simulink library "halout"  (R2021b)
settings: Solver=VariableStepAuto  StartTime=0.0  StopTime=10.0  RelTol=1e-3
undefined symbols (not defined in the file): C_TASK_5MS_S, FALSE, KHAL_CAN1FD1APS3E2E_flg, KHAL_CAN1FD1APS3TxReq_flg, KHAL_CAN1FD1VCU2E2E_flg, KHAL_CAN1FD1VCU2TxReq_flg, KHAL_CAN1FD1VCU3E2E_flg, KHAL_CAN1FD1VCU3TxReq_flg, KHAL_CAN1TxReq_flg, KHAL_CAN1VMCFCM1E2E_flg, KHAL_CAN1VMCFCM1TxReq_flg, KHAL_CAN2TxReq_flg, KHAL_CAN3FD3VCU1toNIDECTxReq_flg, KHAL_CAN3FD3VCU1TxReq_flg, KHAL_CAN3FD3VCU2E2E_flg, KHAL_CAN3FD3VCU2toNIDECE2E_flg, KHAL_CAN3FD3VCU2toNIDECTxReq_flg, KHAL_CAN3FD3VCU2TxReq_flg, KHAL_CAN3TxReq_flg, KHAL_CAN4FD4CE1000E2E_flg, KHAL_CAN4FD4CE1000TxReq_flg, KHAL_CAN4TxReq_flg, KHAL_CAN5TxReq_flg, KHAL_CAN6FD6APS3E2E_flg, KHAL_CAN6FD6APS3TxReq_flg, KHAL_CAN6FD6VCU2E2E_flg, KHAL_CAN6FD6VCU2TxReq_flg, KHAL_CAN6TxReq_flg, ONE_INT, TRUE, ZERO_INT
libraries: FVT_lib x551, simulink x244
(part 1 of 26)
settings Model: Creator=13168  LastModifiedBy=FVT23136
settings SolverCC: AlgebraicLoopSolver=TrustRegion
settings DataIOCC: SaveFormat=Array  SignalLoggingSaveFormat=ModelDataLogs  ReturnWorkspaceOutputs=off
settings OptimizationCC: BlockReduction=off  BooleanDataType=off
settings DebuggingCC: SaveWithParameterizedLinksMsg=none  UnderspecifiedInitializationDetection=Classic  MergeDetectMultiDrivingBlocksExec=none  SignalResolutionControl=TryResolveAllWithWarning  SFMachineParentedDataDiag=warning
settings HardwareCC: TargetUnknown=on
settings ModelReferenceCC: PropagateSignalLabelsOutOfModel=off
settings ConfigComp: CovMetricSettings=dw  CovSaveCumulativeToWorkspaceVar=on  CovSaveSingleToWorkspaceVar=on

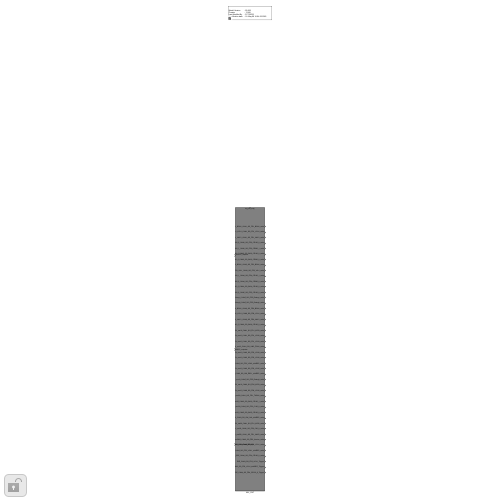
[thumbnail: Simulink's stored preview of the top-level diagram]
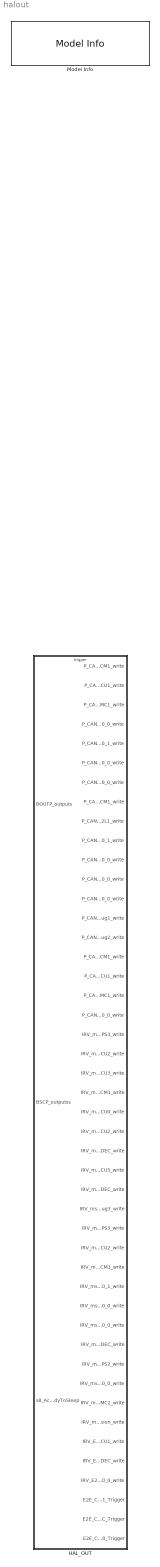
== system halout ==
  HAL_OUT : Subsystem
      settings: RTWSystemCode=Nonreusable function  RTWFcnNameOpts=Use subsystem name  RTWFileNameOpts=Use subsystem name
  Model Info : simulink/Model-Wide Utilities/Model Info  Frame=on  DisplayStringWithTags=|  HorizontalTextAlignment=Left  LeftAlignmentValue=0.02
      | Model Version        : %<ModelVersion>
      | Creator                   : %<Creator>
      | Last Modified By    : %<LastModifiedBy>
      | Modification date    : %<LastModificationDate>

== system halout/HAL_OUT ==
  BOUTP_outputs : Inport  OutDataTypeStr=Bus: BOUTP_outputs
  BSCP_outputss : Inport  Port=2  OutDataTypeStr=Bus: BSCP_outputs
  s8_AcoreReadyToSleep : Inport  Port=3
  trig_hal_out : TriggerPort  TriggerType=function-call  VariantControl=(inherit)
  Bus Selector : BusSelector  OutputSignals=VOUTP_AllCANTxReq_flg
  CAN1 : Subsystem  TreatAsAtomicUnit=on
  CAN2 : Subsystem  TreatAsAtomicUnit=on
  CAN3 : Subsystem  TreatAsAtomicUnit=on
  CAN4 : Subsystem  TreatAsAtomicUnit=on
  CAN5 : Subsystem  TreatAsAtomicUnit=on
  CAN6 : Subsystem  TreatAsAtomicUnit=on
  CAN_Scheduler : Stateflow chart  TreatAsAtomicUnit=on
  Constant : Constant  Value=KHAL_CAN1TxReq_flg
  Constant1 : Constant  Value=KHAL_CAN2TxReq_flg
  Constant2 : Constant  Value=KHAL_CAN3TxReq_flg
  Constant3 : Constant  Value=KHAL_CAN4TxReq_flg
  Constant4 : Constant  Value=KHAL_CAN5TxReq_flg
  Constant5 : Constant  Value=KHAL_CAN6TxReq_flg
  P_CAN1_FD1_BCM1_CAN1_SG_FD1_BCM1_write : Outport  OutDataTypeStr=Bus: DT_CAN1_SG_FD1_BCM1
  P_CAN1_FD1_VCU1_CAN1_SG_FD1_VCU1_write : Outport  Port=2  OutDataTypeStr=Bus: DT_CAN1_SG_FD1_VCU1
  P_CAN1_FD1_VMC1_CAN1_SG_FD1_VMC1_write : Outport  Port=3  OutDataTypeStr=Bus: DT_CAN1_SG_FD1_VMC1
  P_CAN2_FD2_CE100_0_CAN2_SG_FD2_CE100_0_write : Outport  Port=4  OutDataTypeStr=Bus: DT_CAN2_SG_FD2_CE100_0
  P_CAN2_FD2_CE200_1_CAN2_SG_FD2_CE200_1_write : Outport  Port=5  OutDataTypeStr=Bus: DT_CAN2_SG_FD2_CE200_1
  P_CAN2_GW2_CE100_0_CAN2_SG_GW2_CE100_0_write : Outport  Port=6  OutDataTypeStr=Bus: DT_CAN2_SG_GW2_CE100_0
  P_CAN2_GW2_CE200_0_CAN2_SG_GW2_CE200_0_write : Outport  Port=7  OutDataTypeStr=Bus: DT_CAN2_SG_GW2_CE200_0
  P_CAN3_FD3_BCM1_CAN3_SG_FD3_BCM1_write : Outport  Port=8  OutDataTypeStr=Bus: DT_CAN3_SG_FD3_BCM1
  P_CAN3_FD3_V2L1_CAN3_SG_FD3_V2L1_write : Outport  Port=9  OutDataTypeStr=Bus: DT_CAN3_SG_FD3_V2L1
  P_CAN4_FD4_CE100_1_CAN4_SG_FD4_CE100_1_write : Outport  Port=10  OutDataTypeStr=Bus: DT_CAN4_SG_FD4_CE100_1
  P_CAN4_FD4_CE200_0_CAN4_SG_FD4_CE200_0_write : Outport  Port=11  OutDataTypeStr=Bus: DT_CAN4_SG_FD4_CE200_0
  P_CAN4_GW4_CE100_0_CAN4_SG_GW4_CE100_0_write : Outport  Port=12  OutDataTypeStr=Bus: DT_CAN4_SG_GW4_CE100_0
  P_CAN5_FD5_CE100_0_CAN5_SG_FD5_CE100_0_write : Outport  Port=13  OutDataTypeStr=Bus: DT_CAN5_SG_FD5_CE100_0
  P_CAN5_FD5_Debug1_CAN5_SG_FD5_Debug1_write : Outport  Port=14  OutDataTypeStr=Bus: DT_CAN5_SG_FD5_Debug1
  P_CAN5_FD5_Debug2_CAN5_SG_FD5_Debug2_write : Outport  Port=15  OutDataTypeStr=Bus: DT_CAN5_SG_FD5_Debug2
  P_CAN6_FD6_BCM1_CAN6_SG_FD6_BCM1_write : Outport  Port=16  OutDataTypeStr=Bus: DT_CAN6_SG_FD6_BCM1
  P_CAN6_FD6_VCU1_CAN6_SG_FD6_VCU1_write : Outport  Port=17  OutDataTypeStr=Bus: DT_CAN6_SG_FD6_VCU1
  P_CAN6_FD6_VMC1_CAN6_SG_FD6_VMC1_write : Outport  Port=18  OutDataTypeStr=Bus: DT_CAN6_SG_FD6_VMC1
  P_CAN6_GW6_CE100_0_CAN6_SG_GW6_CE100_0_write : Outport  Port=19  OutDataTypeStr=Bus: DT_CAN6_SG_GW6_CE100_0
  IRV_ms10_CAN1_SG_FD1_APS3_write : Outport  Port=20  OutDataTypeStr=Bus: DT_CAN1_SG_FD1_APS3
  IRV_ms10_CAN1_SG_FD1_VCU2_write : Outport  Port=21  OutDataTypeStr=Bus: DT_CAN1_SG_FD1_VCU2
  IRV_ms10_CAN1_SG_FD1_VCU3_write : Outport  Port=22  OutDataTypeStr=Bus: DT_CAN1_SG_FD1_VCU3
  IRV_ms10_CAN1_SG_VMC_FCM1_write : Outport  Port=23  OutDataTypeStr=Bus: DT_CAN1_SG_VMC_FCM1
  IRV_ms10_CAN3_SG_FD3_VCU0_write : Outport  Port=24  OutDataTypeStr=Bus: DT_CAN3_SG_FD3_VCU0
  IRV_ms10_CAN3_SG_FD3_VCU2_write : Outport  Port=25  OutDataTypeStr=Bus: DT_CAN3_SG_FD3_VCU2
  IRV_ms10_CAN3_SG_FD3_VCU2_toNIDEC_write : Outport  Port=26  OutDataTypeStr=Bus: DT_CAN3_SG_FD3_VCU2_toNIDEC
  IRV_ms10_CAN3_SG_FD3_VCU5_write : Outport  Port=27  OutDataTypeStr=Bus: DT_CAN3_SG_FD3_VCU5
  IRV_ms10_CAN3_SG_GW_ESC1_toNIDEC_write : Outport  Port=28  OutDataTypeStr=Bus: DT_CAN3_SG_GW_ESC1_toNIDEC
  IRV_ms10_CAN5_SG_FD5_Debug3_write : Outport  Port=29  OutDataTypeStr=Bus: DT_CAN5_SG_FD5_Debug3
  IRV_ms10_CAN6_SG_FD6_APS3_write : Outport  Port=30  OutDataTypeStr=Bus: DT_CAN6_SG_FD6_APS3
  IRV_ms10_CAN6_SG_FD6_VCU2_write : Outport  Port=31  OutDataTypeStr=Bus: DT_CAN6_SG_FD6_VCU2
  IRV_ms100_CAN1_SG_FD1_THCM1_write : Outport  Port=32  OutDataTypeStr=Bus: DT_CAN1_SG_FD1_THCM1
  IRV_ms100_CAN2_SG_GW2_CE100_1_write : Outport  Port=33  OutDataTypeStr=Bus: DT_CAN2_SG_GW2_CE100_1
  IRV_ms100_CAN3_SG_FD3_C100_0_write : Outport  Port=34  OutDataTypeStr=Bus: DT_CAN3_SG_FD3_C100_0
  IRV_ms100_CAN5_SG_GW5_CE100_0_write : Outport  Port=35  OutDataTypeStr=Bus: DT_CAN5_SG_GW5_CE100_0
  IRV_ms1000_CAN3_SG_GW_IVI6_toNIDEC_write : Outport  Port=36  OutDataTypeStr=Bus: DT_CAN3_SG_GW_IVI6_toNIDEC
  IRV_ms20_CAN1_SG_FD1_APS2_write : Outport  Port=37  OutDataTypeStr=Bus: DT_CAN1_SG_FD1_APS2
  IRV_ms20_CAN2_SG_FD2_C20_0_write : Outport  Port=38  OutDataTypeStr=Bus: DT_CAN2_SG_FD2_C20_0
  IRV_ms500_CAN1_SG_FD1_VMC2_write : Outport  Port=39  OutDataTypeStr=Bus: DT_CAN1_SG_FD1_VMC2
  IRV_ms5000_CAN2_SG_FD2_Version_write : Outport  Port=40  OutDataTypeStr=Bus: DT_CAN2_SG_FD2_Version
  IRV_E2E_CAN3_SG_FD3_VCU1_write : Outport  Port=41  OutDataTypeStr=Bus: DT_CAN3_SG_FD3_VCU1
  IRV_E2E_CAN3_SG_FD3_VCU1_toNIDEC_write : Outport  Port=42  OutDataTypeStr=Bus: DT_CAN3_SG_FD3_VCU1_toNIDEC
  IRV_E2E_CAN4_SG_FD4_CE100_0_write : Outport  Port=43  OutDataTypeStr=Bus: DT_CAN4_SG_FD4_CE100_0
  E2E_CAN3_SG_FD3_VCU1_Trigger : Outport  Port=44
  E2E_CAN3_SG_FD3_VCU1_toNIDEC_Trigger : Outport  Port=45
  E2E_CAN4_SG_FD4_CE100_0_Trigger : Outport  Port=46
  wires:
  BSCP_outputss/1 -> [BSCP_outputs]
  BOUTP_outputs/1 -> [BOUTP_outputs]
  Bus Selector/1 -> CAN_Scheduler/7(VOUTP_ALLCANTxReq_flg)  "<VOUTP_AllCANTxReq_flg>"
  [BOUTP_outputs] -> Bus Selector/1
  Constant1/1 -> CAN_Scheduler/2(KHAL_CAN2TxReq_flg)
  Constant3/1 -> CAN_Scheduler/4(KHAL_CAN4TxReq_flg)
  CAN_Scheduler/1(trig_can1()) -> [trig_can1]
  CAN_Scheduler/2(trig_can2()) -> [trig_can2]
  Constant/1 -> CAN_Scheduler/1(KHAL_CAN1TxReq_flg)
  CAN_Scheduler/4(trig_can4()) -> [trig_can4]
  CAN_Scheduler/5(trig_can5()) -> [trig_can5]
  Constant4/1 -> CAN_Scheduler/5(KHAL_CAN5TxReq_flg)
  Constant2/1 -> CAN_Scheduler/3(KHAL_CAN3TxReq_flg)
  CAN_Scheduler/3(trig_can3()) -> [trig_can3]
  [trig_can1] -> CAN1/Trigger
  [trig_can4] -> CAN4/Trigger
  [trig_can5] -> CAN5/Trigger
  [trig_can2] -> CAN2/Trigger
  Constant5/1 -> CAN_Scheduler/6(KHAL_CAN6TxReq_flg)
  CAN_Scheduler/6(trig_can6()) -> [trig_can6]
  [trig_can6] -> CAN6/Trigger
  [trig_can3] -> CAN3/Trigger
  [BSCP_outputs] -> CAN6/2(BSCP_outputs)
  [BSCP_outputs] -> CAN5/2(BSCP_outputs)
  [BOUTP_outputs] -> CAN5/1(BOUTP_outputs)
  [BOUTP_outputs] -> CAN6/1(BOUTP_outputs)
  CAN4/1(E2E_CAN4_SG_FD4_CE100_0_Trigger) -> E2E_CAN4_SG_FD4_CE100_0_Trigger/1
  [BSCP_outputs] -> CAN3/2(BSCP_outputs)
  CAN3/7(E2E_CAN3_SG_FD3_VCU1_toNIDEC_Trigger) -> E2E_CAN3_SG_FD3_VCU1_toNIDEC_Trigger/1
  [BSCP_outputs] -> CAN2/2(BSCP_outputs)
  [BOUTP_outputs] -> CAN1/1(BOUTP_outputs)
  [BOUTP_outputs] -> CAN3/1(BOUTP_outputs)
  CAN4/2(DT_CAN4_SG_FD4_CE100_0) -> IRV_E2E_CAN4_SG_FD4_CE100_0_write/1
  CAN2/4(DT_CAN2_SG_FD2_Version) -> IRV_ms5000_CAN2_SG_FD2_Version_write/1
  CAN3/8(DT_CAN3_SG_FD3_VCU1_toNIDEC) -> IRV_E2E_CAN3_SG_FD3_VCU1_toNIDEC_write/1
  CAN1/9(DT_CAN1_SG_FD1_VMC2) -> IRV_ms500_CAN1_SG_FD1_VMC2_write/1
  CAN2/1(DT_CAN2_SG_FD2_C20_0) -> IRV_ms20_CAN2_SG_FD2_C20_0_write/1
  CAN1/1(DT_CAN1_SG_FD1_APS2) -> IRV_ms20_CAN1_SG_FD1_APS2_write/1
  CAN3/13(DT_CAN3_SG_GW_IVI6_toNIDEC) -> IRV_ms1000_CAN3_SG_GW_IVI6_toNIDEC_write/1
  CAN5/5(DT_CAN5_SG_GW5_CE100_0) -> IRV_ms100_CAN5_SG_GW5_CE100_0_write/1
  CAN6/4(DT_CAN6_SG_FD6_VCU2) -> IRV_ms10_CAN6_SG_FD6_VCU2_write/1
  CAN5/4(DT_CAN5_SG_FD5_Debug3) -> IRV_ms10_CAN5_SG_FD5_Debug3_write/1
  CAN3/11(DT_CAN3_SG_FD3_VCU5) -> IRV_ms10_CAN3_SG_FD3_VCU5_write/1
  CAN3/12(DT_CAN3_SG_GW_ESC1_toNIDEC) -> IRV_ms10_CAN3_SG_GW_ESC1_toNIDEC_write/1
  CAN2/6(DT_CAN2_SG_GW2_CE100_1) -> IRV_ms100_CAN2_SG_GW2_CE100_1_write/1
  CAN3/10(DT_CAN3_SG_FD3_VCU2_toNIDEC) -> IRV_ms10_CAN3_SG_FD3_VCU2_toNIDEC_write/1
  CAN3/9(DT_CAN3_SG_FD3_VCU2) -> IRV_ms10_CAN3_SG_FD3_VCU2_write/1
  CAN3/4(DT_CAN3_SG_FD3_VCU0) -> IRV_ms10_CAN3_SG_FD3_VCU0_write/1
  CAN1/7(DT_CAN1_SG_FD1_VCU3) -> IRV_ms10_CAN1_SG_FD1_VCU3_write/1
  CAN1/10(DT_CAN1_SG_VMC_FCM1) -> IRV_ms10_CAN1_SG_VMC_FCM1_write/1
  CAN6/5(DT_CAN6_SG_FD6_VMC1) -> P_CAN6_FD6_VMC1_CAN6_SG_FD6_VMC1_write/1
  CAN3/2(DT_CAN3_SG_FD3_C100_0) -> IRV_ms100_CAN3_SG_FD3_C100_0_write/1
  CAN3/5(E2E_CAN3_SG_FD3_VCU1_Trigger) -> E2E_CAN3_SG_FD3_VCU1_Trigger/1
  CAN6/6(DT_CAN6_SG_GW6_CE100_0) -> P_CAN6_GW6_CE100_0_CAN6_SG_GW6_CE100_0_write/1
  CAN1/6(DT_CAN1_SG_FD1_VCU2) -> IRV_ms10_CAN1_SG_FD1_VCU2_write/1
  CAN6/3(DT_CAN6_SG_FD6_VCU1) -> P_CAN6_FD6_VCU1_CAN6_SG_FD6_VCU1_write/1
  CAN6/2(DT_CAN6_SG_FD6_BCM1) -> P_CAN6_FD6_BCM1_CAN6_SG_FD6_BCM1_write/1
  CAN5/2(DT_CAN5_SG_FD5_Debug1) -> P_CAN5_FD5_Debug1_CAN5_SG_FD5_Debug1_write/1
  s8_AcoreReadyToSleep/1 -> CAN3/3(s8_AcoreReadyToSleep)
  CAN5/3(DT_CAN5_SG_FD5_Debug2) -> P_CAN5_FD5_Debug2_CAN5_SG_FD5_Debug2_write/1
  CAN5/1(DT_CAN5_SG_FD5_CE100_0) -> P_CAN5_FD5_CE100_0_CAN5_SG_FD5_CE100_0_write/1
  [BOUTP_outputs] -> CAN4/1(BOUTP_outputs)
  CAN4/5(DT_CAN4_SG_GW4_CE100_0) -> P_CAN4_GW4_CE100_0_CAN4_SG_GW4_CE100_0_write/1
  CAN4/3(DT_CAN4_SG_FD4_CE100_1) -> P_CAN4_FD4_CE100_1_CAN4_SG_FD4_CE100_1_write/1
  CAN4/4(DT_CAN4_SG_FD4_CE200_0) -> P_CAN4_FD4_CE200_0_CAN4_SG_FD4_CE200_0_write/1
  CAN3/3(DT_CAN3_SG_FD3_V2L1) -> P_CAN3_FD3_V2L1_CAN3_SG_FD3_V2L1_write/1
  CAN1/4(DT_CAN1_SG_FD1_THCM1) -> IRV_ms100_CAN1_SG_FD1_THCM1_write/1
  CAN3/1(DT_CAN3_SG_FD3_BCM1) -> P_CAN3_FD3_BCM1_CAN3_SG_FD3_BCM1_write/1
  CAN2/7(DT_CAN2_SG_GW2_CE200_0) -> P_CAN2_GW2_CE200_0_CAN2_SG_GW2_CE200_0_write/1
  CAN1/3(DT_CAN1_SG_FD1_BCM1) -> P_CAN1_FD1_BCM1_CAN1_SG_FD1_BCM1_write/1
  CAN2/5(DT_CAN2_SG_GW2_CE100_0) -> P_CAN2_GW2_CE100_0_CAN2_SG_GW2_CE100_0_write/1
  CAN1/8(DT_CAN1_SG_FD1_VMC1) -> P_CAN1_FD1_VMC1_CAN1_SG_FD1_VMC1_write/1
  CAN1/2(DT_CAN1_SG_FD1_APS3) -> IRV_ms10_CAN1_SG_FD1_APS3_write/1
  [BOUTP_outputs] -> CAN2/1(BOUTP_outputs)
  CAN2/2(DT_CAN2_SG_FD2_CE100_0) -> P_CAN2_FD2_CE100_0_CAN2_SG_FD2_CE100_0_write/1
  CAN6/1(DT_CAN6_SG_FD6_APS3) -> IRV_ms10_CAN6_SG_FD6_APS3_write/1
  CAN1/5(DT_CAN1_SG_FD1_VCU1) -> P_CAN1_FD1_VCU1_CAN1_SG_FD1_VCU1_write/1
  [BSCP_outputs] -> CAN4/2(BSCP_outputs)
  CAN3/6(DT_CAN3_SG_FD3_VCU1) -> IRV_E2E_CAN3_SG_FD3_VCU1_write/1
  CAN2/3(DT_CAN2_SG_FD2_CE200_1) -> P_CAN2_FD2_CE200_1_CAN2_SG_FD2_CE200_1_write/1
  [BSCP_outputs] -> CAN1/2(BSCP_outputs)

== system halout/HAL_OUT/CAN1 ==
  BOUTP_outputs : Inport  OutDataTypeStr=Bus: BOUTP_outputs
  BSCP_outputs : Inport  Port=2  OutDataTypeStr=Bus: BSCP_outputs
  Trigger : TriggerPort  TriggerType=function-call  VariantControl=(inherit)
  Constant : Constant  Value=KHAL_CAN1FD1APS3TxReq_flg
  Constant1 : Constant  Value=KHAL_CAN1FD1VCU2TxReq_flg
  Constant2 : Constant  Value=KHAL_CAN1FD1VCU3TxReq_flg
  Constant3 : Constant  Value=KHAL_CAN1VMCFCM1TxReq_flg
  FD1_APS2_0x210 : Subsystem
  FD1_APS3_0x238 : Subsystem  TreatAsAtomicUnit=on
  FD1_APS3_Tx : Subsystem  AncestorBlock=FVT_lib/hal/MsgTxController  mask{CycleTime=10}
      mask prompts: CycleTime "MsgCycleTime_ms"
      mask help: MeasumentTrigerTime
      mask Display: fprintf('Tx Method: Cycle\nMsg Cycletime ms: %3.0f', CycleTime);
  FD1_BCM1_0x216 : Subsystem
  FD1_THCM1_0x182 : Subsystem
  FD1_VCU1_0x116 : Subsystem
  FD1_VCU2_0x154 : Subsystem  TreatAsAtomicUnit=on
  FD1_VCU2_Tx : Subsystem  AncestorBlock=FVT_lib/hal/MsgTxController  mask{CycleTime=10}
      mask prompts: CycleTime "MsgCycleTime_ms"
      mask help: MeasumentTrigerTime
      mask Display: fprintf('Tx Method: Cycle\nMsg Cycletime ms: %3.0f', CycleTime);
  FD1_VCU3_0x159 : Subsystem  TreatAsAtomicUnit=on
  FD1_VCU3_Tx : Subsystem  AncestorBlock=FVT_lib/hal/MsgTxController  mask{CycleTime=10}
      mask prompts: CycleTime "MsgCycleTime_ms"
      mask help: MeasumentTrigerTime
      mask Display: fprintf('Tx Method: Cycle\nMsg Cycletime ms: %3.0f', CycleTime);
  FD1_VMC1_0x17F : Subsystem
  FD1_VMC2_0x77 : Subsystem
  VMC_FCM1_0x172 : Subsystem  TreatAsAtomicUnit=on
  VMC_FCM1_Tx : Subsystem  AncestorBlock=FVT_lib/hal/MsgTxController  mask{CycleTime=10}
      mask prompts: CycleTime "MsgCycleTime_ms"
      mask help: MeasumentTrigerTime
      mask Display: fprintf('Tx Method: Cycle\nMsg Cycletime ms: %3.0f', CycleTime);
  DT_CAN1_SG_FD1_APS2 : Outport  OutDataTypeStr=Bus: DT_CAN1_SG_FD1_APS2
  DT_CAN1_SG_FD1_APS3 : Outport  Port=2  OutDataTypeStr=Bus: DT_CAN1_SG_FD1_APS3
  DT_CAN1_SG_FD1_BCM1 : Outport  Port=3  OutDataTypeStr=Bus: DT_CAN1_SG_FD1_BCM1
  DT_CAN1_SG_FD1_THCM1 : Outport  Port=4  OutDataTypeStr=Bus: DT_CAN1_SG_FD1_THCM1
  DT_CAN1_SG_FD1_VCU1 : Outport  Port=5  OutDataTypeStr=Bus: DT_CAN1_SG_FD1_VCU1
  DT_CAN1_SG_FD1_VCU2 : Outport  Port=6  OutDataTypeStr=Bus: DT_CAN1_SG_FD1_VCU2
  DT_CAN1_SG_FD1_VCU3 : Outport  Port=7  OutDataTypeStr=Bus: DT_CAN1_SG_FD1_VCU3
  DT_CAN1_SG_FD1_VMC1 : Outport  Port=8  OutDataTypeStr=Bus: DT_CAN1_SG_FD1_VMC1
  DT_CAN1_SG_FD1_VMC2 : Outport  Port=9  OutDataTypeStr=Bus: DT_CAN1_SG_FD1_VMC2
  DT_CAN1_SG_VMC_FCM1 : Outport  Port=10  OutDataTypeStr=Bus: DT_CAN1_SG_VMC_FCM1
  wires:
  BOUTP_outputs/1 -> [BOUTP_outputs]
  BSCP_outputs/1 -> [BSCP_outputs]
  [BSCP_outputs] -> FD1_APS2_0x210/1(BSCP_outputs)
  [BOUTP_outputs] -> FD1_APS2_0x210/2(BOUTP_outputs)
  FD1_APS2_0x210/1(FD1_APS2) -> DT_CAN1_SG_FD1_APS2/1
  [BSCP_outputs] -> FD1_APS3_0x238/1(BSCP_outputs)
  [BOUTP_outputs] -> FD1_APS3_0x238/2(BOUTP_outputs)
  FD1_APS3_Tx/1(TxTrigger) -> FD1_APS3_0x238/Trigger
  Constant/1 -> FD1_APS3_Tx/1(TxReq)
  FD1_APS3_0x238/1(FD1_APS3) -> DT_CAN1_SG_FD1_APS3/1
  [BSCP_outputs] -> FD1_BCM1_0x216/1(BSCP_outputs)
  [BOUTP_outputs] -> FD1_BCM1_0x216/2(BOUTP_outputs)
  FD1_BCM1_0x216/1(FD1_BCM1) -> DT_CAN1_SG_FD1_BCM1/1
  [BSCP_outputs] -> FD1_THCM1_0x182/1(BSCP_outputs)
  [BOUTP_outputs] -> FD1_THCM1_0x182/2(BOUTP_outputs)
  FD1_THCM1_0x182/1(FD1_THCM1) -> DT_CAN1_SG_FD1_THCM1/1
  [BSCP_outputs] -> FD1_VCU1_0x116/1(BSCP_outputs)
  [BOUTP_outputs] -> FD1_VCU1_0x116/2(BOUTP_outputs)
  FD1_VCU1_0x116/1(FD1_VCU1) -> DT_CAN1_SG_FD1_VCU1/1
  [BSCP_outputs] -> FD1_VCU2_0x154/1(BSCP_outputs)
  [BOUTP_outputs] -> FD1_VCU2_0x154/2(BOUTP_outputs)
  FD1_VCU2_Tx/1(TxTrigger) -> FD1_VCU2_0x154/Trigger
  Constant1/1 -> FD1_VCU2_Tx/1(TxReq)
  FD1_VCU2_0x154/1(FD1_VCU2) -> DT_CAN1_SG_FD1_VCU2/1
  [BSCP_outputs] -> FD1_VCU3_0x159/1(BSCP_outputs)
  [BOUTP_outputs] -> FD1_VCU3_0x159/2(BOUTP_outputs)
  FD1_VCU3_Tx/1(TxTrigger) -> FD1_VCU3_0x159/Trigger
  Constant2/1 -> FD1_VCU3_Tx/1(TxReq)
  FD1_VCU3_0x159/1(FD1_VCU3) -> DT_CAN1_SG_FD1_VCU3/1
  [BSCP_outputs] -> FD1_VMC1_0x17F/1(BSCP_outputs)
  [BOUTP_outputs] -> FD1_VMC1_0x17F/2(BOUTP_outputs)
  FD1_VMC1_0x17F/1(FD1_VMC1) -> DT_CAN1_SG_FD1_VMC1/1
  [BSCP_outputs] -> FD1_VMC2_0x77/1(BSCP_outputs)
  [BOUTP_outputs] -> FD1_VMC2_0x77/2(BOUTP_outputs)
  FD1_VMC2_0x77/1(FD1_VMC2) -> DT_CAN1_SG_FD1_VMC2/1
  [BSCP_outputs] -> VMC_FCM1_0x172/1(BSCP_outputs)
  [BOUTP_outputs] -> VMC_FCM1_0x172/2(BOUTP_outputs)
  VMC_FCM1_Tx/1(TxTrigger) -> VMC_FCM1_0x172/Trigger
  Constant3/1 -> VMC_FCM1_Tx/1(TxReq)
  VMC_FCM1_0x172/1(VMC_FCM1) -> DT_CAN1_SG_VMC_FCM1/1

== system halout/HAL_OUT/CAN2 ==
  BOUTP_outputs : Inport  OutDataTypeStr=Bus: BOUTP_outputs
  BSCP_outputs : Inport  Port=2  OutDataTypeStr=Bus: BSCP_outputs
  Trigger : TriggerPort  TriggerType=function-call  VariantControl=(inherit)
  FD2_C20_0_0x210 : Subsystem
  FD2_CE100_0_0x117 : Subsystem
  FD2_CE200_1_0x435 : Subsystem
  FD2_Version_0x3C3 : Subsystem
  GW2_CE100_0_0x1C2 : Subsystem
  GW2_CE100_1_0x357 : Subsystem
  GW2_CE200_0_0x174 : Subsystem
  DT_CAN2_SG_FD2_C20_0 : Outport  OutDataTypeStr=Bus: DT_CAN2_SG_FD2_C20_0
  DT_CAN2_SG_FD2_CE100_0 : Outport  Port=2  OutDataTypeStr=Bus: DT_CAN2_SG_FD2_CE100_0
  DT_CAN2_SG_FD2_CE200_1 : Outport  Port=3  OutDataTypeStr=Bus: DT_CAN2_SG_FD2_CE200_1
  DT_CAN2_SG_FD2_Version : Outport  Port=4  OutDataTypeStr=Bus: DT_CAN2_SG_FD2_Version
  DT_CAN2_SG_GW2_CE100_0 : Outport  Port=5  OutDataTypeStr=Bus: DT_CAN2_SG_GW2_CE100_0
  DT_CAN2_SG_GW2_CE100_1 : Outport  Port=6  OutDataTypeStr=Bus: DT_CAN2_SG_GW2_CE100_1
  DT_CAN2_SG_GW2_CE200_0 : Outport  Port=7  OutDataTypeStr=Bus: DT_CAN2_SG_GW2_CE200_0
  wires:
  BOUTP_outputs/1 -> [BOUTP_outputs]
  BSCP_outputs/1 -> [BSCP_outputs]
  [BSCP_outputs] -> FD2_C20_0_0x210/1(BSCP_outputs)
  [BOUTP_outputs] -> FD2_C20_0_0x210/2(BOUTP_outputs)
  FD2_C20_0_0x210/1(FD2_C20_0) -> DT_CAN2_SG_FD2_C20_0/1
  [BSCP_outputs] -> FD2_CE100_0_0x117/1(BSCP_outputs)
  [BOUTP_outputs] -> FD2_CE100_0_0x117/2(BOUTP_outputs)
  FD2_CE100_0_0x117/1(FD2_CE100_0) -> DT_CAN2_SG_FD2_CE100_0/1
  [BSCP_outputs] -> FD2_CE200_1_0x435/1(BSCP_outputs)
  [BOUTP_outputs] -> FD2_CE200_1_0x435/2(BOUTP_outputs)
  FD2_CE200_1_0x435/1(FD2_CE200_1) -> DT_CAN2_SG_FD2_CE200_1/1
  [BSCP_outputs] -> FD2_Version_0x3C3/1(BSCP_outputs)
  [BOUTP_outputs] -> FD2_Version_0x3C3/2(BOUTP_outputs)
  FD2_Version_0x3C3/1(FD2_Version) -> DT_CAN2_SG_FD2_Version/1
  [BSCP_outputs] -> GW2_CE100_0_0x1C2/1(BSCP_outputs)
  [BOUTP_outputs] -> GW2_CE100_0_0x1C2/2(BOUTP_outputs)
  GW2_CE100_0_0x1C2/1(GW2_CE100_0) -> DT_CAN2_SG_GW2_CE100_0/1
  [BSCP_outputs] -> GW2_CE100_1_0x357/1(BSCP_outputs)
  [BOUTP_outputs] -> GW2_CE100_1_0x357/2(BOUTP_outputs)
  GW2_CE100_1_0x357/1(GW2_CE100_1) -> DT_CAN2_SG_GW2_CE100_1/1
  [BSCP_outputs] -> GW2_CE200_0_0x174/1(BSCP_outputs)
  [BOUTP_outputs] -> GW2_CE200_0_0x174/2(BOUTP_outputs)
  GW2_CE200_0_0x174/1(GW2_CE200_0) -> DT_CAN2_SG_GW2_CE200_0/1

== system halout/HAL_OUT/CAN3 ==
  BOUTP_outputs : Inport  OutDataTypeStr=Bus: BOUTP_outputs
  BSCP_outputs : Inport  Port=2  OutDataTypeStr=Bus: BSCP_outputs
  s8_AcoreReadyToSleep : Inport  Port=3
  Trigger : TriggerPort  TriggerType=function-call  VariantControl=(inherit)
  Constant : Constant  Value=KHAL_CAN3FD3VCU1TxReq_flg
  Constant1 : Constant  Value=KHAL_CAN3FD3VCU1toNIDECTxReq_flg
  Constant2 : Constant  Value=KHAL_CAN3FD3VCU2TxReq_flg
  Constant3 : Constant  Value=KHAL_CAN3FD3VCU2toNIDECTxReq_flg
  FD3_BCM1_0x216 : Subsystem
  FD3_C100_0_0x182 : Subsystem
  FD3_V2L1_0x374 : Subsystem
  FD3_VCU0_0x1F0 : Subsystem
  FD3_VCU1_0x115 : Subsystem
  FD3_VCU1_Tx : Subsystem  AncestorBlock=FVT_lib/hal/MsgTxController_CE  mask{CycleTime=100}
      mask prompts: CycleTime "MsgCycleTime_ms"
      mask help: MeasumentTrigerTime
      mask Display: fprintf('Tx Method: CE\nMsg Cycletime ms: %3.0f', CycleTime);
  FD3_VCU1_toNIDEC_0x116 : Subsystem
  FD3_VCU1_toNIDEC_Tx : Subsystem  AncestorBlock=FVT_lib/hal/MsgTxController_CE  mask{CycleTime=100}
      mask prompts: CycleTime "MsgCycleTime_ms"
      mask help: MeasumentTrigerTime
      mask Display: fprintf('Tx Method: CE\nMsg Cycletime ms: %3.0f', CycleTime);
  FD3_VCU2_0x153 : Subsystem  TreatAsAtomicUnit=on
  FD3_VCU2_Tx : Subsystem  AncestorBlock=FVT_lib/hal/MsgTxController  mask{CycleTime=10}
      mask prompts: CycleTime "MsgCycleTime_ms"
      mask help: MeasumentTrigerTime
      mask Display: fprintf('Tx Method: Cycle\nMsg Cycletime ms: %3.0f', CycleTime);
  FD3_VCU2_toNIDEC_0x154 : Subsystem  TreatAsAtomicUnit=on
  FD3_VCU2_toNIDEC_Tx : Subsystem  AncestorBlock=FVT_lib/hal/MsgTxController  mask{CycleTime=10}
      mask prompts: CycleTime "MsgCycleTime_ms"
      mask help: MeasumentTrigerTime
      mask Display: fprintf('Tx Method: Cycle\nMsg Cycletime ms: %3.0f', CycleTime);
  FD3_VCU5_0x155 : Subsystem
  GW_ESC1_toNIDEC_0x152 : Subsystem
  GW_IVI6_toNIDEC_0x49F : Subsystem
  DT_CAN3_SG_FD3_BCM1 : Outport  OutDataTypeStr=Bus: DT_CAN3_SG_FD3_BCM1
  DT_CAN3_SG_FD3_C100_0 : Outport  Port=2  OutDataTypeStr=Bus: DT_CAN3_SG_FD3_C100_0
  DT_CAN3_SG_FD3_V2L1 : Outport  Port=3  OutDataTypeStr=Bus: DT_CAN3_SG_FD3_V2L1
  DT_CAN3_SG_FD3_VCU0 : Outport  Port=4  OutDataTypeStr=Bus: DT_CAN3_SG_FD3_VCU0
  E2E_CAN3_SG_FD3_VCU1_Trigger : Outport  Port=5
  DT_CAN3_SG_FD3_VCU1 : Outport  Port=6  OutDataTypeStr=Bus: DT_CAN3_SG_FD3_VCU1
  E2E_CAN3_SG_FD3_VCU1_toNIDEC_Trigger : Outport  Port=7
  DT_CAN3_SG_FD3_VCU1_toNIDEC : Outport  Port=8  OutDataTypeStr=Bus: DT_CAN3_SG_FD3_VCU1_toNIDEC
  DT_CAN3_SG_FD3_VCU2 : Outport  Port=9  OutDataTypeStr=Bus: DT_CAN3_SG_FD3_VCU2
  DT_CAN3_SG_FD3_VCU2_toNIDEC : Outport  Port=10  OutDataTypeStr=Bus: DT_CAN3_SG_FD3_VCU2_toNIDEC
  DT_CAN3_SG_FD3_VCU5 : Outport  Port=11  OutDataTypeStr=Bus: DT_CAN3_SG_FD3_VCU5
  DT_CAN3_SG_GW_ESC1_toNIDEC : Outport  Port=12  OutDataTypeStr=Bus: DT_CAN3_SG_GW_ESC1_toNIDEC
  DT_CAN3_SG_GW_IVI6_toNIDEC : Outport  Port=13  OutDataTypeStr=Bus: DT_CAN3_SG_GW_IVI6_toNIDEC
  wires:
  BOUTP_outputs/1 -> [BOUTP_outputs]
  BSCP_outputs/1 -> [BSCP_outputs]
  [BSCP_outputs] -> FD3_BCM1_0x216/1(BSCP_outputs)
  [BOUTP_outputs] -> FD3_BCM1_0x216/2(BOUTP_outputs)
  FD3_BCM1_0x216/1(FD3_BCM1) -> DT_CAN3_SG_FD3_BCM1/1
  [BSCP_outputs] -> FD3_C100_0_0x182/1(BSCP_outputs)
  [BOUTP_outputs] -> FD3_C100_0_0x182/2(BOUTP_outputs)
  FD3_C100_0_0x182/1(FD3_C100_0) -> DT_CAN3_SG_FD3_C100_0/1
  [BSCP_outputs] -> FD3_V2L1_0x374/1(BSCP_outputs)
  [BOUTP_outputs] -> FD3_V2L1_0x374/2(BOUTP_outputs)
  FD3_V2L1_0x374/1(FD3_V2L1) -> DT_CAN3_SG_FD3_V2L1/1
  [BSCP_outputs] -> FD3_VCU0_0x1F0/1(BSCP_outputs)
  [BOUTP_outputs] -> FD3_VCU0_0x1F0/2(BOUTP_outputs)
  FD3_VCU0_0x1F0/1(FD3_VCU0) -> DT_CAN3_SG_FD3_VCU0/1
  [BSCP_outputs] -> FD3_VCU1_0x115/1(BSCP_outputs)
  [BOUTP_outputs] -> FD3_VCU1_0x115/2(BOUTP_outputs)
  FD3_VCU1_Tx/1(TxTrigger) -> E2E_CAN3_SG_FD3_VCU1_Trigger/1
  Constant/1 -> FD3_VCU1_Tx/1(TxReq)
  [BSCP_outputs] -> FD3_VCU1_Tx/2(BSCP_outputs)
  [BOUTP_outputs] -> FD3_VCU1_Tx/3(BOUTP_outputs)
  FD3_VCU1_0x115/1(FD3_VCU1) -> DT_CAN3_SG_FD3_VCU1/1
  [BSCP_outputs] -> FD3_VCU1_toNIDEC_0x116/1(BSCP_outputs)
  [BOUTP_outputs] -> FD3_VCU1_toNIDEC_0x116/2(BOUTP_outputs)
  FD3_VCU1_toNIDEC_Tx/1(TxTrigger) -> E2E_CAN3_SG_FD3_VCU1_toNIDEC_Trigger/1
  Constant1/1 -> FD3_VCU1_toNIDEC_Tx/1(TxReq)
  [BSCP_outputs] -> FD3_VCU1_toNIDEC_Tx/2(BSCP_outputs)
  [BOUTP_outputs] -> FD3_VCU1_toNIDEC_Tx/3(BOUTP_outputs)
  FD3_VCU1_toNIDEC_0x116/1(FD3_VCU1_toNIDEC) -> DT_CAN3_SG_FD3_VCU1_toNIDEC/1
  [BSCP_outputs] -> FD3_VCU2_0x153/1(BSCP_outputs)
  [BOUTP_outputs] -> FD3_VCU2_0x153/2(BOUTP_outputs)
  FD3_VCU2_Tx/1(TxTrigger) -> FD3_VCU2_0x153/Trigger
  Constant2/1 -> FD3_VCU2_Tx/1(TxReq)
  FD3_VCU2_0x153/1(FD3_VCU2) -> DT_CAN3_SG_FD3_VCU2/1
  [BSCP_outputs] -> FD3_VCU2_toNIDEC_0x154/1(BSCP_outputs)
  [BOUTP_outputs] -> FD3_VCU2_toNIDEC_0x154/2(BOUTP_outputs)
  FD3_VCU2_toNIDEC_Tx/1(TxTrigger) -> FD3_VCU2_toNIDEC_0x154/Trigger
  Constant3/1 -> FD3_VCU2_toNIDEC_Tx/1(TxReq)
  FD3_VCU2_toNIDEC_0x154/1(FD3_VCU2_toNIDEC) -> DT_CAN3_SG_FD3_VCU2_toNIDEC/1
  [BSCP_outputs] -> FD3_VCU5_0x155/1(BSCP_outputs)
  [BOUTP_outputs] -> FD3_VCU5_0x155/2(BOUTP_outputs)
  FD3_VCU5_0x155/1(FD3_VCU5) -> DT_CAN3_SG_FD3_VCU5/1
  [BSCP_outputs] -> GW_ESC1_toNIDEC_0x152/1(BSCP_outputs)
  [BOUTP_outputs] -> GW_ESC1_toNIDEC_0x152/2(BOUTP_outputs)
  GW_ESC1_toNIDEC_0x152/1(GW_ESC1_toNIDEC) -> DT_CAN3_SG_GW_ESC1_toNIDEC/1
  [BSCP_outputs] -> GW_IVI6_toNIDEC_0x49F/1(BSCP_outputs)
  [BOUTP_outputs] -> GW_IVI6_toNIDEC_0x49F/2(BOUTP_outputs)
  GW_IVI6_toNIDEC_0x49F/1(GW_IVI6_toNIDEC) -> DT_CAN3_SG_GW_IVI6_toNIDEC/1
  s8_AcoreReadyToSleep/1 -> FD3_VCU0_0x1F0/3(s8_AcoreReadyToSleep)

== system halout/HAL_OUT/CAN4 ==
  BOUTP_outputs : Inport  OutDataTypeStr=Bus: BOUTP_outputs
  BSCP_outputs : Inport  Port=2  OutDataTypeStr=Bus: BSCP_outputs
  Trigger : TriggerPort  TriggerType=function-call  VariantControl=(inherit)
  Constant : Constant  Value=KHAL_CAN4FD4CE1000TxReq_flg
  Detect Change : simulink/Logic and Bit Operations/Detect Change  vinit=0  OutDataTypeStr=boolean
  FD4_CE100_0_0x116 : Subsystem  TreatAsAtomicUnit=on
  FD4_CE100_0_Tx : Subsystem  AncestorBlock=FVT_lib/hal/MsgTxController_CE  mask{CycleTime=100}
      mask prompts: CycleTime "MsgCycleTime_ms"
      mask help: MeasumentTrigerTime
      mask Display: fprintf('Tx Method: CE\nMsg Cycletime ms: %3.0f', CycleTime);
  FD4_CE100_1_0x182 : Subsystem
  FD4_CE200_0_0x217 : Subsystem
  Function-Call Subsystem : Subsystem  TreatAsAtomicUnit=on
  GW4_CE100_0_0x253 : Subsystem
  Unit Delay : UnitDelay  SampleTime=-1  HasFrameUpgradeWarning=on
  E2E_CAN4_SG_FD4_CE100_0_Trigger : Outport
  DT_CAN4_SG_FD4_CE100_0 : Outport  Port=2  OutDataTypeStr=Bus: DT_CAN4_SG_FD4_CE100_0
  DT_CAN4_SG_FD4_CE100_1 : Outport  Port=3  OutDataTypeStr=Bus: DT_CAN4_SG_FD4_CE100_1
  DT_CAN4_SG_FD4_CE200_0 : Outport  Port=4  OutDataTypeStr=Bus: DT_CAN4_SG_FD4_CE200_0
  DT_CAN4_SG_GW4_CE100_0 : Outport  Port=5  OutDataTypeStr=Bus: DT_CAN4_SG_GW4_CE100_0
  wires:
  BOUTP_outputs/1 -> [BOUTP_outputs]
  BSCP_outputs/1 -> [BSCP_outputs]
  [BSCP_outputs] -> FD4_CE100_0_0x116/1(BSCP_outputs)
  [BOUTP_outputs] -> FD4_CE100_0_0x116/2(BOUTP_outputs)
  Constant/1 -> FD4_CE100_0_Tx/1(TxReq)
  [BSCP_outputs] -> FD4_CE100_0_Tx/2(BSCP_outputs)
  [BOUTP_outputs] -> FD4_CE100_0_Tx/3(BOUTP_outputs)
  FD4_CE100_0_0x116/1(FD4_CE100_0) -> DT_CAN4_SG_FD4_CE100_0/1
  [BSCP_outputs] -> FD4_CE100_1_0x182/1(BSCP_outputs)
  [BOUTP_outputs] -> FD4_CE100_1_0x182/2(BOUTP_outputs)
  FD4_CE100_1_0x182/1(FD4_CE100_1) -> DT_CAN4_SG_FD4_CE100_1/1
  [BSCP_outputs] -> FD4_CE200_0_0x217/1(BSCP_outputs)
  [BOUTP_outputs] -> FD4_CE200_0_0x217/2(BOUTP_outputs)
  FD4_CE200_0_0x217/1(FD4_CE200_0) -> DT_CAN4_SG_FD4_CE200_0/1
  [BSCP_outputs] -> GW4_CE100_0_0x253/1(BSCP_outputs)
  [BOUTP_outputs] -> GW4_CE100_0_0x253/2(BOUTP_outputs)
  GW4_CE100_0_0x253/1(GW4_CE100_0) -> DT_CAN4_SG_GW4_CE100_0/1
  Detect Change/1 -> Unit Delay/1
  Function-Call Subsystem/1(TriggerCAN4VCU1_CNT) -> Detect Change/1
  Unit Delay/1 -> E2E_CAN4_SG_FD4_CE100_0_Trigger/1
  FD4_CE100_0_Tx/1(TxTrigger) -> FD4_CE100_0_0x116/Trigger
  FD4_CE100_0_Tx/2(TriggerCallCDD) -> Function-Call Subsystem/Trigger

== system halout/HAL_OUT/CAN5 ==
  BOUTP_outputs : Inport  OutDataTypeStr=Bus: BOUTP_outputs
  BSCP_outputs : Inport  Port=2  OutDataTypeStr=Bus: BSCP_outputs
  Trigger : TriggerPort  TriggerType=function-call  VariantControl=(inherit)
  FD5_CE100_0_0x118 : Subsystem
  FD5_Debug1_0x4D0 : Subsystem
  FD5_Debug2_0x4F7 : Subsystem
  FD5_Debug3_0x4F3 : Subsystem
  GW5_CE100_0_0x1C5 : Subsystem
  DT_CAN5_SG_FD5_CE100_0 : Outport  OutDataTypeStr=Bus: DT_CAN5_SG_FD5_CE100_0
  DT_CAN5_SG_FD5_Debug1 : Outport  Port=2  OutDataTypeStr=Bus: DT_CAN5_SG_FD5_Debug1
  DT_CAN5_SG_FD5_Debug2 : Outport  Port=3  OutDataTypeStr=Bus: DT_CAN5_SG_FD5_Debug2
  DT_CAN5_SG_FD5_Debug3 : Outport  Port=4  OutDataTypeStr=Bus: DT_CAN5_SG_FD5_Debug3
  DT_CAN5_SG_GW5_CE100_0 : Outport  Port=5  OutDataTypeStr=Bus: DT_CAN5_SG_GW5_CE100_0
  wires:
  BOUTP_outputs/1 -> [BOUTP_outputs]
  BSCP_outputs/1 -> [BSCP_outputs]
  [BSCP_outputs] -> FD5_CE100_0_0x118/1(BSCP_outputs)
  [BOUTP_outputs] -> FD5_CE100_0_0x118/2(BOUTP_outputs)
  FD5_CE100_0_0x118/1(FD5_CE100_0) -> DT_CAN5_SG_FD5_CE100_0/1
  [BSCP_outputs] -> FD5_Debug1_0x4D0/1(BSCP_outputs)
  [BOUTP_outputs] -> FD5_Debug1_0x4D0/2(BOUTP_outputs)
  FD5_Debug1_0x4D0/1(FD5_Debug1) -> DT_CAN5_SG_FD5_Debug1/1
  [BSCP_outputs] -> FD5_Debug2_0x4F7/1(BSCP_outputs)
  [BOUTP_outputs] -> FD5_Debug2_0x4F7/2(BOUTP_outputs)
  FD5_Debug2_0x4F7/1(FD5_Debug2) -> DT_CAN5_SG_FD5_Debug2/1
  [BSCP_outputs] -> FD5_Debug3_0x4F3/1(BSCP_outputs)
  [BOUTP_outputs] -> FD5_Debug3_0x4F3/2(BOUTP_outputs)
  FD5_Debug3_0x4F3/1(FD5_Debug3) -> DT_CAN5_SG_FD5_Debug3/1
  [BSCP_outputs] -> GW5_CE100_0_0x1C5/1(BSCP_outputs)
  [BOUTP_outputs] -> GW5_CE100_0_0x1C5/2(BOUTP_outputs)
  GW5_CE100_0_0x1C5/1(GW5_CE100_0) -> DT_CAN5_SG_GW5_CE100_0/1

== system halout/HAL_OUT/CAN6 ==
  BOUTP_outputs : Inport  OutDataTypeStr=Bus: BOUTP_outputs
  BSCP_outputs : Inport  Port=2  OutDataTypeStr=Bus: BSCP_outputs
  Trigger : TriggerPort  TriggerType=function-call  VariantControl=(inherit)
  Constant : Constant  Value=KHAL_CAN6FD6APS3TxReq_flg
  Constant1 : Constant  Value=KHAL_CAN6FD6VCU2TxReq_flg
  FD6_APS3_0x238 : Subsystem  TreatAsAtomicUnit=on
  FD6_APS3_Tx : Subsystem  AncestorBlock=FVT_lib/hal/MsgTxController  mask{CycleTime=10}
      mask prompts: CycleTime "MsgCycleTime_ms"
      mask help: MeasumentTrigerTime
      mask Display: fprintf('Tx Method: Cycle\nMsg Cycletime ms: %3.0f', CycleTime);
  FD6_BCM1_0x216 : Subsystem
  FD6_VCU1_0x116 : Subsystem
  FD6_VCU2_0x154 : Subsystem  TreatAsAtomicUnit=on
  FD6_VCU2_Tx : Subsystem  AncestorBlock=FVT_lib/hal/MsgTxController  mask{CycleTime=10}
      mask prompts: CycleTime "MsgCycleTime_ms"
      mask help: MeasumentTrigerTime
      mask Display: fprintf('Tx Method: Cycle\nMsg Cycletime ms: %3.0f', CycleTime);
  FD6_VMC1_0x17F : Subsystem
  GW6_CE100_0_0x1C6 : Subsystem
  DT_CAN6_SG_FD6_APS3 : Outport  OutDataTypeStr=Bus: DT_CAN6_SG_FD6_APS3
  DT_CAN6_SG_FD6_BCM1 : Outport  Port=2  OutDataTypeStr=Bus: DT_CAN6_SG_FD6_BCM1
  DT_CAN6_SG_FD6_VCU1 : Outport  Port=3  OutDataTypeStr=Bus: DT_CAN6_SG_FD6_VCU1
  DT_CAN6_SG_FD6_VCU2 : Outport  Port=4  OutDataTypeStr=Bus: DT_CAN6_SG_FD6_VCU2
  DT_CAN6_SG_FD6_VMC1 : Outport  Port=5  OutDataTypeStr=Bus: DT_CAN6_SG_FD6_VMC1
  DT_CAN6_SG_GW6_CE100_0 : Outport  Port=6  OutDataTypeStr=Bus: DT_CAN6_SG_GW6_CE100_0
  wires:
  BOUTP_outputs/1 -> [BOUTP_outputs]
  BSCP_outputs/1 -> [BSCP_outputs]
  [BSCP_outputs] -> FD6_APS3_0x238/1(BSCP_outputs)
  [BOUTP_outputs] -> FD6_APS3_0x238/2(BOUTP_outputs)
  FD6_APS3_Tx/1(TxTrigger) -> FD6_APS3_0x238/Trigger
  Constant/1 -> FD6_APS3_Tx/1(TxReq)
  FD6_APS3_0x238/1(FD6_APS3) -> DT_CAN6_SG_FD6_APS3/1
  [BSCP_outputs] -> FD6_BCM1_0x216/1(BSCP_outputs)
  [BOUTP_outputs] -> FD6_BCM1_0x216/2(BOUTP_outputs)
  FD6_BCM1_0x216/1(FD6_BCM1) -> DT_CAN6_SG_FD6_BCM1/1
  [BSCP_outputs] -> FD6_VCU1_0x116/1(BSCP_outputs)
  [BOUTP_outputs] -> FD6_VCU1_0x116/2(BOUTP_outputs)
  FD6_VCU1_0x116/1(FD6_VCU1) -> DT_CAN6_SG_FD6_VCU1/1
  [BSCP_outputs] -> FD6_VCU2_0x154/1(BSCP_outputs)
  [BOUTP_outputs] -> FD6_VCU2_0x154/2(BOUTP_outputs)
  FD6_VCU2_Tx/1(TxTrigger) -> FD6_VCU2_0x154/Trigger
  Constant1/1 -> FD6_VCU2_Tx/1(TxReq)
  FD6_VCU2_0x154/1(FD6_VCU2) -> DT_CAN6_SG_FD6_VCU2/1
  [BSCP_outputs] -> FD6_VMC1_0x17F/1(BSCP_outputs)
  [BOUTP_outputs] -> FD6_VMC1_0x17F/2(BOUTP_outputs)
  FD6_VMC1_0x17F/1(FD6_VMC1) -> DT_CAN6_SG_FD6_VMC1/1
  [BSCP_outputs] -> GW6_CE100_0_0x1C6/1(BSCP_outputs)
  [BOUTP_outputs] -> GW6_CE100_0_0x1C6/2(BOUTP_outputs)
  GW6_CE100_0_0x1C6/1(GW6_CE100_0) -> DT_CAN6_SG_GW6_CE100_0/1

== system halout/HAL_OUT/CAN1/FD1_APS2_0x210 ==
  BSCP_outputs : Inport  OutDataTypeStr=Bus: BSCP_outputs
  BOUTP_outputs : Inport  Port=2  OutDataTypeStr=Bus: BOUTP_outputs
  APSDFLL : Subsystem
  APSDFLR : Subsystem
  APSDRLL : Subsystem
  APSDRLR : Subsystem
  APSExitCondition : Subsystem
  APSHWVer : Subsystem
  APSProgressPCT : Subsystem
  APSRQDisplay : Subsystem
  APSSWVer : Subsystem
  PASAFCL : Subsystem
  PASAFCR : Subsystem
  PASAFML : Subsystem
  PASAFMR : Subsystem
  PASARCL : Subsystem
  PASARCR : Subsystem
  PASARML : Subsystem
  PASARMR : Subsystem
  PASChime : Subsystem
  PASDFCL : Subsystem
  PASDFCR : Subsystem
  PASDFML : Subsystem
  PASDFMR : Subsystem
  PASDRCL : Subsystem
  PASDRCR : Subsystem
  PASDRML : Subsystem
  PASDRMR : Subsystem
  PASModOperation : Subsystem
  PASSNSRLayout : Subsystem
  PASStaFSys : Subsystem
  USSStaFCL : Subsystem
  USSStaFCR : Subsystem
  USSStaFLL : Subsystem
  USSStaFLR : Subsystem
  USSStaFML : Subsystem
  USSStaFMR : Subsystem
  USSStaRCL : Subsystem
  USSStaRCR : Subsystem
  USSStaRLL : Subsystem
  USSStaRLR : Subsystem
  USSStaRML : Subsystem
  USSStaRMR : Subsystem
  bus_creator : BusCreator  Inputs=41  OutDataTypeStr=Bus: DT_CAN1_SG_FD1_APS2  NonVirtualBus=on
  bus_selector : BusSelector  OutputSignals=VOUTP_APSDFLL_cm
  bus_selector1 : BusSelector  OutputSignals=VOUTP_APSDFLR_cm
  bus_selector10 : BusSelector  OutputSignals=VOUTP_PASAFCR_enum
  bus_selector11 : BusSelector  OutputSignals=VOUTP_PASAFML_enum
  bus_selector12 : BusSelector  OutputSignals=VOUTP_PASAFMR_enum
  bus_selector13 : BusSelector  OutputSignals=VOUTP_PASARCL_enum
  bus_selector14 : BusSelector  OutputSignals=VOUTP_PASARCR_enum
  bus_selector15 : BusSelector  OutputSignals=VOUTP_PASARML_enum
  bus_selector16 : BusSelector  OutputSignals=VOUTP_PASARMR_enum
  bus_selector17 : BusSelector  OutputSignals=VOUTP_Chime_enum
  bus_selector18 : BusSelector  OutputSignals=VOUTP_PASDFCL_cm
  bus_selector19 : BusSelector  OutputSignals=VOUTP_PASDFCR_cm
  bus_selector2 : BusSelector  OutputSignals=VOUTP_APSDRLL_cm
  bus_selector20 : BusSelector  OutputSignals=VOUTP_PASDFML_cm
  bus_selector21 : BusSelector  OutputSignals=VOUTP_PASDFMR_cm
  bus_selector22 : BusSelector  OutputSignals=VOUTP_PASDRCL_cm
  bus_selector23 : BusSelector  OutputSignals=VOUTP_PASDRCR_cm
  bus_selector24 : BusSelector  OutputSignals=VOUTP_PASDRML_cm
  bus_selector25 : BusSelector  OutputSignals=VOUTP_PASDRMR_cm
  bus_selector26 : BusSelector  OutputSignals=VOUTP_ModOperation_enum
  bus_selector27 : BusSelector  OutputSignals=VOUTP_SNSRLayout_enum
  bus_selector28 : BusSelector  OutputSignals=VOUTP_StaFSya_flg
  bus_selector29 : BusSelector  OutputSignals=VOUTP_USSStaFCL_flg
  bus_selector3 : BusSelector  OutputSignals=VOUTP_APSDRLR_cm
  bus_selector30 : BusSelector  OutputSignals=VOUTP_USSStaFCR_flg
  bus_selector31 : BusSelector  OutputSignals=VOUTP_USSStaFLL_flg
  bus_selector32 : BusSelector  OutputSignals=VOUTP_USSStaFLR_flg
  bus_selector33 : BusSelector  OutputSignals=VOUTP_USSStaFML_flg
  bus_selector34 : BusSelector  OutputSignals=VOUTP_USSStaFMR_flg
  bus_selector35 : BusSelector  OutputSignals=VOUTP_USSStaRCL_flg
  bus_selector36 : BusSelector  OutputSignals=VOUTP_USSStaRCR_flg
  bus_selector37 : BusSelector  OutputSignals=VOUTP_USSStaRLL_flg
  bus_selector38 : BusSelector  OutputSignals=VOUTP_USSStaRLR_flg
  bus_selector39 : BusSelector  OutputSignals=VOUTP_USSStaRML_flg
  bus_selector4 : BusSelector  OutputSignals=VOUTP_APSExitCondition_enum
  bus_selector40 : BusSelector  OutputSignals=VOUTP_USSStaRMR_flg
  bus_selector5 : BusSelector  OutputSignals=VOUTP_APSHWVer_enum
  bus_selector6 : BusSelector  OutputSignals=VOUTP_APSProgressPCT_pct
  bus_selector7 : BusSelector  OutputSignals=VOUTP_APSRQDisplay_enum
  bus_selector8 : BusSelector  OutputSignals=VOUTP_APSSWVer_enum
  bus_selector9 : BusSelector  OutputSignals=VOUTP_PASAFCL_enum
  FD1_APS2 : Outport
  wires:
  BSCP_outputs/1 -> [BSCP_outputs]
  BOUTP_outputs/1 -> [BOUTP_outputs]
  [CAN1_APS_D_FLL] -> bus_creator/1  "CAN1_APS_D_FLL"
  [CAN1_APS_D_FLR] -> bus_creator/2  "CAN1_APS_D_FLR"
  [CAN1_APS_D_RLL] -> bus_creator/3  "CAN1_APS_D_RLL"
  [CAN1_APS_D_RLR] -> bus_creator/4  "CAN1_APS_D_RLR"
  [CAN1_APS_ExitCondition] -> bus_creator/5  "CAN1_APS_ExitCondition"
  [CAN1_APS_HW_Ver] -> bus_creator/6  "CAN1_APS_HW_Ver"
  [CAN1_APS_Progress_PCT] -> bus_creator/7  "CAN1_APS_Progress_PCT"
  [CAN1_APS_RQ_Display] -> bus_creator/8  "CAN1_APS_RQ_Display"
  [CAN1_APS_SW_Ver] -> bus_creator/9  "CAN1_APS_SW_Ver"
  [CAN1_PAS_A_FCL] -> bus_creator/10  "CAN1_PAS_A_FCL"
  [CAN1_PAS_A_FCR] -> bus_creator/11  "CAN1_PAS_A_FCR"
  [CAN1_PAS_A_FML] -> bus_creator/12  "CAN1_PAS_A_FML"
  [CAN1_PAS_A_FMR] -> bus_creator/13  "CAN1_PAS_A_FMR"
  [CAN1_PAS_A_RCL] -> bus_creator/14  "CAN1_PAS_A_RCL"
  [CAN1_PAS_A_RCR] -> bus_creator/15  "CAN1_PAS_A_RCR"
  [CAN1_PAS_A_RML] -> bus_creator/16  "CAN1_PAS_A_RML"
  [CAN1_PAS_A_RMR] -> bus_creator/17  "CAN1_PAS_A_RMR"
  [CAN1_PAS_Chime] -> bus_creator/18  "CAN1_PAS_Chime"
  [CAN1_PAS_D_FCL] -> bus_creator/19  "CAN1_PAS_D_FCL"
  [CAN1_PAS_D_FCR] -> bus_creator/20  "CAN1_PAS_D_FCR"
  [CAN1_PAS_D_FML] -> bus_creator/21  "CAN1_PAS_D_FML"
  [CAN1_PAS_D_FMR] -> bus_creator/22  "CAN1_PAS_D_FMR"
  [CAN1_PAS_D_RCL] -> bus_creator/23  "CAN1_PAS_D_RCL"
  [CAN1_PAS_D_RCR] -> bus_creator/24  "CAN1_PAS_D_RCR"
  [CAN1_PAS_D_RML] -> bus_creator/25  "CAN1_PAS_D_RML"
  [CAN1_PAS_D_RMR] -> bus_creator/26  "CAN1_PAS_D_RMR"
  [CAN1_PAS_Mod_Operation] -> bus_creator/27  "CAN1_PAS_Mod_Operation"
  [CAN1_PAS_SNSR_Layout] -> bus_creator/28  "CAN1_PAS_SNSR_Layout"
  [CAN1_PAS_Sta_F_Sys] -> bus_creator/29  "CAN1_PAS_Sta_F_Sys"
  [CAN1_USS_Sta_FCL] -> bus_creator/30  "CAN1_USS_Sta_FCL"
  [CAN1_USS_Sta_FCR] -> bus_creator/31  "CAN1_USS_Sta_FCR"
  [CAN1_USS_Sta_FLL] -> bus_creator/32  "CAN1_USS_Sta_FLL"
  [CAN1_USS_Sta_FLR] -> bus_creator/33  "CAN1_USS_Sta_FLR"
  [CAN1_USS_Sta_FML] -> bus_creator/34  "CAN1_USS_Sta_FML"
  [CAN1_USS_Sta_FMR] -> bus_creator/35  "CAN1_USS_Sta_FMR"
  [CAN1_USS_Sta_RCL] -> bus_creator/36  "CAN1_USS_Sta_RCL"
  [CAN1_USS_Sta_RCR] -> bus_creator/37  "CAN1_USS_Sta_RCR"
  [CAN1_USS_Sta_RLL] -> bus_creator/38  "CAN1_USS_Sta_RLL"
  [CAN1_USS_Sta_RLR] -> bus_creator/39  "CAN1_USS_Sta_RLR"
  [CAN1_USS_Sta_RML] -> bus_creator/40  "CAN1_USS_Sta_RML"
  [CAN1_USS_Sta_RMR] -> bus_creator/41  "CAN1_USS_Sta_RMR"
  bus_creator/1 -> FD1_APS2/1
  APSDFLL/1(CAN1_APS_D_FLL) -> [CAN1_APS_D_FLL]
  APSDFLR/1(CAN1_APS_D_FLR) -> [CAN1_APS_D_FLR]
  APSDRLL/1(CAN1_APS_D_RLL) -> [CAN1_APS_D_RLL]
  APSDRLR/1(CAN1_APS_D_RLR) -> [CAN1_APS_D_RLR]
  APSExitCondition/1(CAN1_APS_ExitCondition) -> [CAN1_APS_ExitCondition]
  APSHWVer/1(CAN1_APS_HW_Ver) -> [CAN1_APS_HW_Ver]
  APSProgressPCT/1(CAN1_APS_Progress_PCT) -> [CAN1_APS_Progress_PCT]
  APSRQDisplay/1(CAN1_APS_RQ_Display) -> [CAN1_APS_RQ_Display]
  APSSWVer/1(CAN1_APS_SW_Ver) -> [CAN1_APS_SW_Ver]
  PASAFCL/1(CAN1_PAS_A_FCL) -> [CAN1_PAS_A_FCL]
  PASAFCR/1(CAN1_PAS_A_FCR) -> [CAN1_PAS_A_FCR]
  PASAFML/1(CAN1_PAS_A_FML) -> [CAN1_PAS_A_FML]
  PASAFMR/1(CAN1_PAS_A_FMR) -> [CAN1_PAS_A_FMR]
  PASARCL/1(CAN1_PAS_A_RCL) -> [CAN1_PAS_A_RCL]
  PASARCR/1(CAN1_PAS_A_RCR) -> [CAN1_PAS_A_RCR]
  PASARML/1(CAN1_PAS_A_RML) -> [CAN1_PAS_A_RML]
  PASARMR/1(CAN1_PAS_A_RMR) -> [CAN1_PAS_A_RMR]
  PASChime/1(CAN1_PAS_Chime) -> [CAN1_PAS_Chime]
  PASDFCL/1(CAN1_PAS_D_FCL) -> [CAN1_PAS_D_FCL]
  PASDFCR/1(CAN1_PAS_D_FCR) -> [CAN1_PAS_D_FCR]
  PASDFML/1(CAN1_PAS_D_FML) -> [CAN1_PAS_D_FML]
  PASDFMR/1(CAN1_PAS_D_FMR) -> [CAN1_PAS_D_FMR]
  PASDRCL/1(CAN1_PAS_D_RCL) -> [CAN1_PAS_D_RCL]
  PASDRCR/1(CAN1_PAS_D_RCR) -> [CAN1_PAS_D_RCR]
  PASDRML/1(CAN1_PAS_D_RML) -> [CAN1_PAS_D_RML]
  PASDRMR/1(CAN1_PAS_D_RMR) -> [CAN1_PAS_D_RMR]
  PASModOperation/1(CAN1_PAS_Mod_Operation) -> [CAN1_PAS_Mod_Operation]
  PASSNSRLayout/1(CAN1_PAS_SNSR_Layout) -> [CAN1_PAS_SNSR_Layout]
  PASStaFSys/1(CAN1_PAS_Sta_F_Sys) -> [CAN1_PAS_Sta_F_Sys]
  USSStaFCL/1(CAN1_USS_Sta_FCL) -> [CAN1_USS_Sta_FCL]
  USSStaFCR/1(CAN1_USS_Sta_FCR) -> [CAN1_USS_Sta_FCR]
  USSStaFLL/1(CAN1_USS_Sta_FLL) -> [CAN1_USS_Sta_FLL]
  USSStaFLR/1(CAN1_USS_Sta_FLR) -> [CAN1_USS_Sta_FLR]
  USSStaFML/1(CAN1_USS_Sta_FML) -> [CAN1_USS_Sta_FML]
  USSStaFMR/1(CAN1_USS_Sta_FMR) -> [CAN1_USS_Sta_FMR]
  USSStaRCL/1(CAN1_USS_Sta_RCL) -> [CAN1_USS_Sta_RCL]
  USSStaRCR/1(CAN1_USS_Sta_RCR) -> [CAN1_USS_Sta_RCR]
  USSStaRLL/1(CAN1_USS_Sta_RLL) -> [CAN1_USS_Sta_RLL]
  USSStaRLR/1(CAN1_USS_Sta_RLR) -> [CAN1_USS_Sta_RLR]
  USSStaRML/1(CAN1_USS_Sta_RML) -> [CAN1_USS_Sta_RML]
  USSStaRMR/1(CAN1_USS_Sta_RMR) -> [CAN1_USS_Sta_RMR]
  bus_selector/1 -> APSDFLL/1(APSDFLL)  "<VOUTP_APSDFLL_cm>"
  [BOUTP_outputs] -> bus_selector/1
  bus_selector1/1 -> APSDFLR/1(APSDFLR)  "<VOUTP_APSDFLR_cm>"
  [BOUTP_outputs] -> bus_selector1/1
  bus_selector2/1 -> APSDRLL/1(APSDRLL)  "<VOUTP_APSDRLL_cm>"
  [BOUTP_outputs] -> bus_selector2/1
  bus_selector3/1 -> APSDRLR/1(APSDRLR)  "<VOUTP_APSDRLR_cm>"
  [BOUTP_outputs] -> bus_selector3/1
  bus_selector4/1 -> APSExitCondition/1(APSExitCondition)  "<VOUTP_APSExitCondition_enum>"
  [BOUTP_outputs] -> bus_selector4/1
  bus_selector5/1 -> APSHWVer/1(APSHWVer)  "<VOUTP_APSHWVer_enum>"
  [BOUTP_outputs] -> bus_selector5/1
  bus_selector6/1 -> APSProgressPCT/1(APSProgressPCT)  "<VOUTP_APSProgressPCT_pct>"
  [BOUTP_outputs] -> bus_selector6/1
  bus_selector7/1 -> APSRQDisplay/1(APSRQDisplay)  "<VOUTP_APSRQDisplay_enum>"
  [BOUTP_outputs] -> bus_selector7/1
  bus_selector8/1 -> APSSWVer/1(APSSWVer)  "<VOUTP_APSSWVer_enum>"
  [BOUTP_outputs] -> bus_selector8/1
  bus_selector9/1 -> PASAFCL/1(PASAFCL)  "<VOUTP_PASAFCL_enum>"
  [BOUTP_outputs] -> bus_selector9/1
  bus_selector10/1 -> PASAFCR/1(PASAFCR)  "<VOUTP_PASAFCR_enum>"
  [BOUTP_outputs] -> bus_selector10/1
  bus_selector11/1 -> PASAFML/1(PASAFML)  "<VOUTP_PASAFML_enum>"
  [BOUTP_outputs] -> bus_selector11/1
  bus_selector12/1 -> PASAFMR/1(PASAFMR)  "<VOUTP_PASAFMR_enum>"
  [BOUTP_outputs] -> bus_selector12/1
  bus_selector13/1 -> PASARCL/1(PASARCL)  "<VOUTP_PASARCL_enum>"
  [BOUTP_outputs] -> bus_selector13/1
  bus_selector14/1 -> PASARCR/1(PASARCR)  "<VOUTP_PASARCR_enum>"
  [BOUTP_outputs] -> bus_selector14/1
  bus_selector15/1 -> PASARML/1(PASARML)  "<VOUTP_PASARML_enum>"
  [BOUTP_outputs] -> bus_selector15/1
  bus_selector16/1 -> PASARMR/1(PASARMR)  "<VOUTP_PASARMR_enum>"
  [BOUTP_outputs] -> bus_selector16/1
  bus_selector17/1 -> PASChime/1(PASChime)  "<VOUTP_Chime_enum>"
  [BOUTP_outputs] -> bus_selector17/1
  bus_selector18/1 -> PASDFCL/1(PASDFCL)  "<VOUTP_PASDFCL_cm>"
  [BOUTP_outputs] -> bus_selector18/1
  bus_selector19/1 -> PASDFCR/1(PASDFCR)  "<VOUTP_PASDFCR_cm>"
  [BOUTP_outputs] -> bus_selector19/1
  bus_selector20/1 -> PASDFML/1(PASDFML)  "<VOUTP_PASDFML_cm>"
  [BOUTP_outputs] -> bus_selector20/1
  bus_selector21/1 -> PASDFMR/1(PASDFMR)  "<VOUTP_PASDFMR_cm>"
  [BOUTP_outputs] -> bus_selector21/1
  bus_selector22/1 -> PASDRCL/1(PASDRCL)  "<VOUTP_PASDRCL_cm>"
  [BOUTP_outputs] -> bus_selector22/1
  bus_selector23/1 -> PASDRCR/1(PASDRCR)  "<VOUTP_PASDRCR_cm>"
  [BOUTP_outputs] -> bus_selector23/1
  bus_selector24/1 -> PASDRML/1(PASDRML)  "<VOUTP_PASDRML_cm>"
  [BOUTP_outputs] -> bus_selector24/1
  bus_selector25/1 -> PASDRMR/1(PASDRMR)  "<VOUTP_PASDRMR_cm>"
  [BOUTP_outputs] -> bus_selector25/1
  bus_selector26/1 -> PASModOperation/1(PASModOperation)  "<VOUTP_ModOperation_enum>"
  [BOUTP_outputs] -> bus_selector26/1
  bus_selector27/1 -> PASSNSRLayout/1(PASSNSRLayout)  "<VOUTP_SNSRLayout_enum>"
  [BOUTP_outputs] -> bus_selector27/1
  bus_selector28/1 -> PASStaFSys/1(PASStaFSys)  "<VOUTP_StaFSya_flg>"
  [BOUTP_outputs] -> bus_selector28/1
  bus_selector29/1 -> USSStaFCL/1(USSStaFCL)  "<VOUTP_USSStaFCL_flg>"
  [BOUTP_outputs] -> bus_selector29/1
  bus_selector30/1 -> USSStaFCR/1(USSStaFCR)  "<VOUTP_USSStaFCR_flg>"
  [BOUTP_outputs] -> bus_selector30/1
  bus_selector31/1 -> USSStaFLL/1(USSStaFLL)  "<VOUTP_USSStaFLL_flg>"
  [BOUTP_outputs] -> bus_selector31/1
  bus_selector32/1 -> USSStaFLR/1(USSStaFLR)  "<VOUTP_USSStaFLR_flg>"
  [BOUTP_outputs] -> bus_selector32/1
  bus_selector33/1 -> USSStaFML/1(USSStaFML)  "<VOUTP_USSStaFML_flg>"
  [BOUTP_outputs] -> bus_selector33/1
  bus_selector34/1 -> USSStaFMR/1(USSStaFMR)  "<VOUTP_USSStaFMR_flg>"
  [BOUTP_outputs] -> bus_selector34/1
  bus_selector35/1 -> USSStaRCL/1(USSStaRCL)  "<VOUTP_USSStaRCL_flg>"
  [BOUTP_outputs] -> bus_selector35/1
  bus_selector36/1 -> USSStaRCR/1(USSStaRCR)  "<VOUTP_USSStaRCR_flg>"
  [BOUTP_outputs] -> bus_selector36/1
  bus_selector37/1 -> USSStaRLL/1(USSStaRLL)  "<VOUTP_USSStaRLL_flg>"
  [BOUTP_outputs] -> bus_selector37/1
  bus_selector38/1 -> USSStaRLR/1(USSStaRLR)  "<VOUTP_USSStaRLR_flg>"
  [BOUTP_outputs] -> bus_selector38/1
  bus_selector39/1 -> USSStaRML/1(USSStaRML)  "<VOUTP_USSStaRML_flg>"
  [BOUTP_outputs] -> bus_selector39/1
  bus_selector40/1 -> USSStaRMR/1(USSStaRMR)  "<VOUTP_USSStaRMR_flg>"
  [BOUTP_outputs] -> bus_selector40/1
